simulink model "subsistema_termico"  (R2020a)
settings: Solver=VariableStepAuto  StartTime=0.0  StopTime=10.0  RelTol=1e-3
model workspace: external: MATLAB File D:\Ferran\Facultad\UNCuyo\Meca\Automática y Máquinas Eléctricas\Proyecto final\matlab2\parametros_y_especs\parametros_y_especif.m (data not in the file)
undefined symbols (not defined in the file): alpha_Cu, Cts, Rref, Rts_amb, Tref
settings Model: Creator=Ferran  LastModifiedBy=Ferran

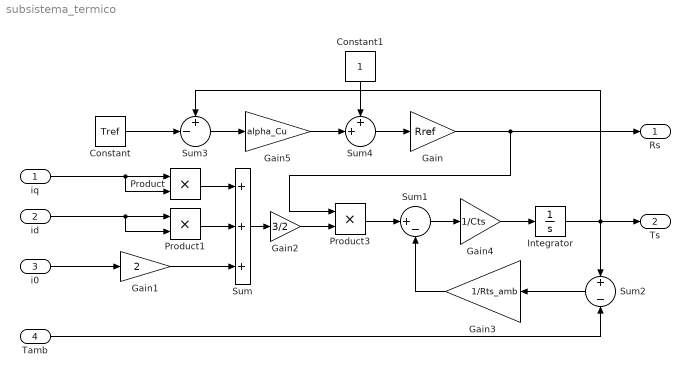
== system subsistema_termico ==
  iq : Inport
  id : Inport  Port=2
  i0 : Inport  Port=3
  Tamb : Inport  Port=4
  Constant : Constant  Value=Tref
  Constant1 : Constant
  Gain : Gain  Gain=Rref
  Gain1 : Gain  Gain=2
  Gain2 : Gain  Gain=3/2
  Gain3 : Gain  Gain=1/Rts_amb
  Gain4 : Gain  Gain=1/Cts
  Gain5 : Gain  Gain=alpha_Cu
  Integrator : Integrator  InitialCondition=20
  Product : Product
  Product1 : Product
  Product3 : Product
  Sum : Sum  Inputs=+++
  Sum1 : Sum  Inputs=|+-
  Sum2 : Sum  Inputs=+-
  Sum3 : Sum  Inputs=+-|
  Sum4 : Sum  Inputs=++|
  Rs : Outport
  Ts : Outport  Port=2
  wires:
  iq/1 -> Product/1, Product/2
  id/1 -> Product1/1, Product1/2
  Product/1 -> Sum/1
  Product1/1 -> Sum/2
  i0/1 -> Gain1/1
  Sum/1 -> Gain2/1
  Gain/1 -> Product3/1, Rs/1
  Product3/1 -> Sum1/1
  Integrator/1 -> Sum3/1, Sum2/1, Ts/1
  Tamb/1 -> Sum2/2
  Sum2/1 -> Gain3/1
  Gain3/1 -> Sum1/2
  Sum1/1 -> Gain4/1
  Gain4/1 -> Integrator/1
  Sum3/1 -> Gain5/1
  Gain5/1 -> Sum4/2
  Constant1/1 -> Sum4/1
  Sum4/1 -> Gain/1
  Constant/1 -> Sum3/2
  Gain1/1 -> Sum/3
  Gain2/1 -> Product3/2
